simulink model "Task"  (R2023a)
settings: Solver=VariableStepAuto  StartTime=0.0  StopTime=10.0  RelTol=1e-3
values from neighbouring files (symbols this model uses):
  A = [-0.435 0.209 0.02 ... (first row only)    [MatlabCode.m]
  B = [1 ... (first row only)    [MatlabCode.m]
  C = [0.0003 0 0]    [MatlabCode.m]
  D = [0]    [MatlabCode.m]
undefined symbols (not defined in the file or in its folder): K, L
settings Model: Creator=aalia  LastModifiedBy=aalia

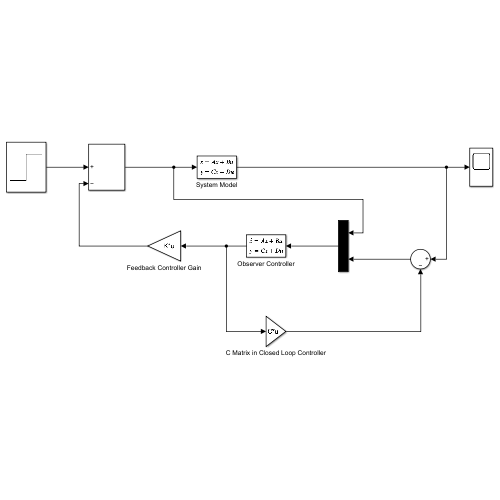
[thumbnail: Simulink's stored preview of the top-level diagram]
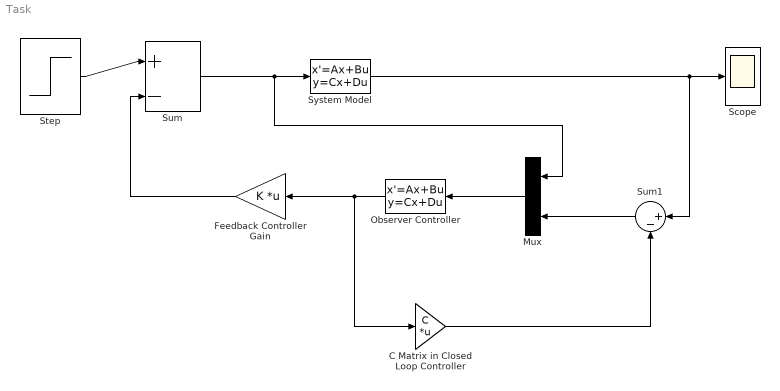
== system Task ==
  C Matrix in Closed Loop Controller : Gain  Gain=C  Multiplication=Matrix(K*u)
  Feedback Controller Gain : Gain  Gain=K  Multiplication=Matrix(K*u)
  Mux : Mux  Inputs=2
  Observer Controller : StateSpace  A=A  B=[B L]  C=[1 0 0; 0 1 0; 0 0 1]  D=[0 0; 0 0; 0 0]  InitialCondition=0
  Scope : Scope
  Step : Step  Time=0  SampleTime=0
  Sum : Sum  Inputs=|+-
  Sum1 : Sum  Inputs=|+-
  System Model : StateSpace  A=A  B=B  C=C  D=D  InitialCondition=0
  wires:
  Step/1 -> Sum/1
  Feedback Controller Gain/1 -> Sum/2
  C Matrix in Closed Loop Controller/1 -> Sum1/2
  Observer Controller/1 -> C Matrix in Closed Loop Controller/1, Feedback Controller Gain/1
  Sum/1 -> Mux/1, System Model/1
  System Model/1 -> Sum1/1, Scope/1
  Sum1/1 -> Mux/2
  Mux/1 -> Observer Controller/1
